simulink model "q4withFWBR"  (R2018a)
settings: Solver=FixedStepAuto  StartTime=0  StopTime=0.6  FixedStep=1e-6  RelTol=1e-3
libraries: powerlib x27, dspstat3 x2
settings Model: Creator=c  LastModifiedBy=asus

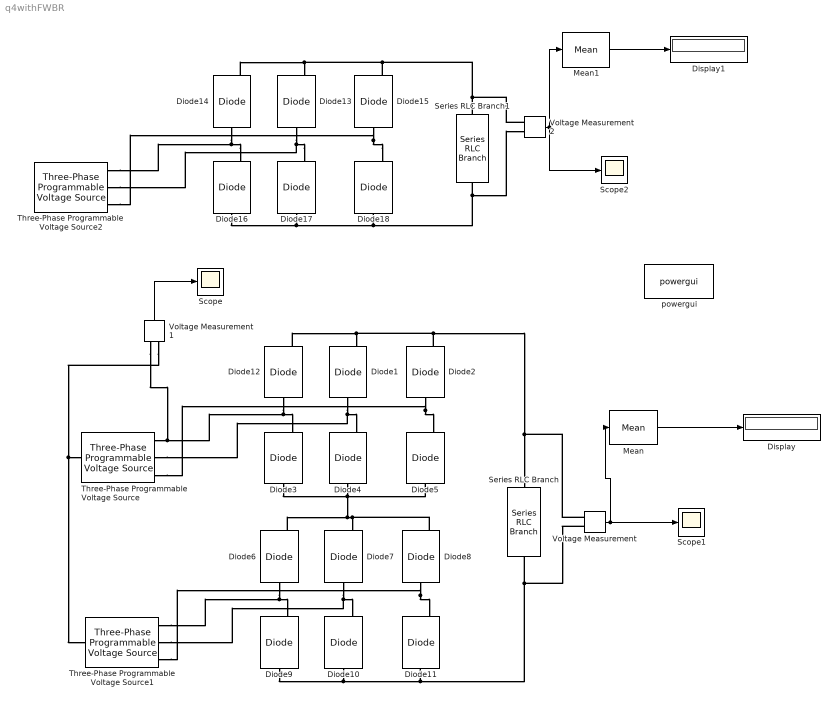
== system q4withFWBR ==
  Diode{1..18} (18 alike) : powerlib/Power Electronics/Diode  Ron=1e-9  Lon=0  Vf=0  IC=0  UseSnubber=0  Rs=500  Cs=250e-9  Measurements=on
  Display : Display
  Display1 : Display
  Mean : dspstat3/Mean  run=off  InputProcessing=Columns as channels (frame based)  reset_popup=None  directionMode=Each column  dimension=1  roiEnable=off  roiType=Rectangles  roiPortion=Entire ROI  roiOutput=Individual statistics for each ROI  roiFlag=off  roundingMode=Floor  overflowMode=off  outputDataTypeStr=Inherit: Same as accumulator  outputMin=[]  outputMax=[]  outputLastDataTypeStr=Inherit: Same as accumulator
  Mean1 : dspstat3/Mean  run=off  InputProcessing=Columns as channels (frame based)  reset_popup=None  directionMode=Each column  dimension=1  roiEnable=off  roiType=Rectangles  roiPortion=Entire ROI  roiOutput=Individual statistics for each ROI  roiFlag=off  roundingMode=Floor  overflowMode=off  outputDataTypeStr=Inherit: Same as accumulator  outputMin=[]  outputMax=[]  outputLastDataTypeStr=Inherit: Same as accumulator
  Scope : Scope
  Scope1 : Scope
  Scope2 : Scope
  Series RLC Branch : powerlib/Elements/Series RLC Branch  LConnTagsString=__new0  RConnTagsString=__new0  BranchType=R  Resistance=10  Inductance=1e-3  SetiL0=off  InitialCurrent=0  Capacitance=1e-6  Setx0=off  InitialVoltage=0  Measurements=None
  Series RLC Branch1 : powerlib/Elements/Series RLC Branch  LConnTagsString=__new0  RConnTagsString=__new0  BranchType=R  Resistance=10  Inductance=1e-3  SetiL0=off  InitialCurrent=0  Capacitance=1e-6  Setx0=off  InitialVoltage=0  Measurements=None
  Three-Phase Programmable Voltage Source : powerlib/Electrical Sources/Three-Phase Programmable Voltage Source  PositiveSequence="[100  0 50]"  VariationEntity=None  VariationType=Table of time-amplitude pairs  VariationTypeAlt=Step  VariationStep=0.5  VariationRate=10  VariationMagnitude=0.3  VariationFrequency=2  VariationTiming=[1 2]  VariationPhaseA=off  Amplitudes=[1 0.8 1.2 1.0]  TimeValues=[0 0.1 0.15 0.2]  HarmonicGeneration=off  HarmonicA=[3 0.2 -25 0]  HarmonicB=[2 0.15 35 2]  Timing="[0.05  3]"  BusType=swing  Pref=0  Qref=0  Qmin=-inf  Qmax=inf
  Three-Phase Programmable Voltage Source1 : powerlib/Electrical Sources/Three-Phase Programmable Voltage Source  PositiveSequence="[100  30 50]"  VariationEntity=None  VariationType=Table of time-amplitude pairs  VariationTypeAlt=Step  VariationStep=0.5  VariationRate=10  VariationMagnitude=0.3  VariationFrequency=2  VariationTiming=[1 2]  VariationPhaseA=off  Amplitudes=[1 0.8 1.2 1.0]  TimeValues=[0 0.1 0.15 0.2]  HarmonicGeneration=off  HarmonicA=[3 0.2 -25 0]  HarmonicB=[2 0.15 35 2]  Timing="[0.05  3]"  BusType=swing  Pref=0  Qref=0  Qmin=-inf  Qmax=inf
  Three-Phase Programmable Voltage Source2 : powerlib/Electrical Sources/Three-Phase Programmable Voltage Source  PositiveSequence="[107.75  0 50]"  VariationEntity=None  VariationType=Table of time-amplitude pairs  VariationTypeAlt=Step  VariationStep=0.5  VariationRate=10  VariationMagnitude=0.3  VariationFrequency=2  VariationTiming=[1 2]  VariationPhaseA=off  Amplitudes=[1 0.8 1.2 1.0]  TimeValues=[0 0.1 0.15 0.2]  HarmonicGeneration=off  HarmonicA=[3 0.2 -25 0]  HarmonicB=[2 0.15 35 2]  Timing="[0.05  3]"  BusType=swing  Pref=0  Qref=0  Qmin=-inf  Qmax=inf
  Voltage Measurement : powerlib/Measurements/Voltage Measurement  PhasorSimulation=off  OutputType=Complex  PSBequivalent=0
  Voltage Measurement1 : powerlib/Measurements/Voltage Measurement  PhasorSimulation=off  OutputType=Complex  PSBequivalent=0
  Voltage Measurement2 : powerlib/Measurements/Voltage Measurement  PhasorSimulation=off  OutputType=Complex  PSBequivalent=0
  powergui : powerlib/powergui  Priority=1  SimulationMode=Discrete  SampleTime=5e-5  frequency=60  Iterations=50  frequencyindice=50  Pbase=100e6  ErrMax=1e-4  UnitsV=kV  UnitsW=MW  buscounter=0  FunctionMessages=off  echomessages=off  EnableUseOfTLC=off  CurrentSourceSwitches=off  DisableSnubberDevices=off  DisableRonSwitches=off  DisableVfSwitches=off  DisplayEquations=off  SolverType=Tustin/Backward Euler (TBE)  Interpol=off  ExternalGateDelay=off  methode=off  Ts=100  x0status=blocks  SPID=off  SwTol=0  HookPort=off  RestoreLinks=warning  ResistiveCurrentMeasurement=off  Frange=[0:2:500]  Ylog=off  Xlog=on  ShowGrid=off  save=off  variable=ZData  structure=0  ZoomFFT=off  StartTime=0.0  cycles=1  DisplayStyle=1  fundamental=60  FreqAxis=off  MaxFrequency=1000  frequencyindicesteady=1  RmsSteady=1  display=off
  wires:
  Voltage Measurement/1 -> Mean/1, Scope1/1
  Mean/1 -> Display/1
  Voltage Measurement1/1 -> Scope/1
  Voltage Measurement2/1 -> Mean1/1, Scope2/1
  Mean1/1 -> Display1/1
  connections:
  Voltage Measurement1/LConn1 -- Three-Phase Programmable Voltage Source/RConn1 -- Diode12/LConn1 -- Diode3/RConn1
  Diode1/LConn1 -- Three-Phase Programmable Voltage Source/RConn2 -- Diode4/RConn1
  Diode2/LConn1 -- Diode5/RConn1 -- Three-Phase Programmable Voltage Source/RConn3
  Diode2/RConn1 -- Voltage Measurement/LConn1 -- Series RLC Branch/LConn1 -- Diode12/RConn1 -- Diode1/RConn1
  Diode6/LConn1 -- Three-Phase Programmable Voltage Source1/RConn1 -- Diode9/RConn1
  Diode9/LConn1 -- Diode10/LConn1 -- Voltage Measurement/LConn2 -- Series RLC Branch/RConn1 -- Diode11/LConn1
  Diode7/LConn1 -- Three-Phase Programmable Voltage Source1/RConn2 -- Diode10/RConn1
  Diode3/LConn1 -- Diode5/LConn1 -- Diode7/RConn1 -- Diode8/RConn1 -- Diode6/RConn1 -- Diode4/LConn1
  Diode8/LConn1 -- Three-Phase Programmable Voltage Source1/RConn3 -- Diode11/RConn1
  Voltage Measurement1/LConn2 -- Three-Phase Programmable Voltage Source1/LConn1 -- Three-Phase Programmable Voltage Source/LConn1
  Diode18/RConn1 -- Three-Phase Programmable Voltage Source2/RConn3 -- Diode15/LConn1
  Series RLC Branch1/LConn1 -- Voltage Measurement2/LConn1 -- Diode15/RConn1 -- Diode14/RConn1 -- Diode13/RConn1
  Diode17/LConn1 -- Diode16/LConn1 -- Diode18/LConn1 -- Voltage Measurement2/LConn2 -- Series RLC Branch1/RConn1
  Diode17/RConn1 -- Three-Phase Programmable Voltage Source2/RConn2 -- Diode13/LConn1
  Diode16/RConn1 -- Three-Phase Programmable Voltage Source2/RConn1 -- Diode14/LConn1
